simulink model "SHIP_DOWN_PT2000_matlab_2017"  (R2018b)
settings: Solver=ode8  StartTime=0.0  StopTime=2.5  RelTol=1e-3
undefined symbols (not defined in the file): Cout_c, Cout_r, Cvh_c, Cvh_r, dellay_f1, dellay_f2, dellay_f3, dellay_f4, dellay_f5, dellay_f6, DiscIntNeverNeededParam, f, L1_l, L1_r, Lvh_l, Lvh_r, R_out, Uout, Uvh
libraries: powerlib x92, simulink x18, simulink_extras x18, powerlib_meascontrol x13
(part 2 of 2)

== system SHIP_DOWN_PT2000_matlab_2017/Силовой блок 2/PWM4 ==
  Uz : Inport
  Data Type Conversion : DataTypeConversion  OutDataTypeStr=boolean
  Delay1 : Delay  DelayLength=dellay_f4  InitialCondition=0  UseCircularBuffer=on
  Logical Operator : Logic  Operator=NOT  AllPortsSameDT=off  OutDataTypeStr=boolean
  Relay1 : Relay  OnSwitchValue=0.01  OffSwitchValue=-0.01
  Repeating Sequence1 : simulink/Sources/Repeating Sequence  rep_seq_t="[0  (1/(2*f)) (1/f)]"  rep_seq_y=[0 1 0]
  S-R Flip-Flop : simulink_extras/Flip Flops/S-R Flip-Flop  initial_condition=0
  Sum : Sum  Inputs=+-
  Terminator : Terminator
  CH1 : Outport
  wires:
  S-R Flip-Flop/1 -> CH1/1
  Data Type Conversion/1 -> S-R Flip-Flop/1
  Logical Operator/1 -> S-R Flip-Flop/2
  Relay1/1 -> Logical Operator/1, Data Type Conversion/1
  Uz/1 -> Sum/1
  Sum/1 -> Relay1/1
  S-R Flip-Flop/2 -> Terminator/1
  Repeating Sequence1/1 -> Delay1/1
  Delay1/1 -> Sum/2

== system SHIP_DOWN_PT2000_matlab_2017/Силовой блок 2/PWM5 ==
  Uz : Inport
  Data Type Conversion : DataTypeConversion  OutDataTypeStr=boolean
  Delay1 : Delay  DelayLength=dellay_f5  InitialCondition=0  UseCircularBuffer=on
  Logical Operator : Logic  Operator=NOT  AllPortsSameDT=off  OutDataTypeStr=boolean
  Relay1 : Relay  OnSwitchValue=0.01  OffSwitchValue=-0.01
  Repeating Sequence1 : simulink/Sources/Repeating Sequence  rep_seq_t="[0  (1/(2*f)) (1/f)]"  rep_seq_y=[0 1 0]
  S-R Flip-Flop : simulink_extras/Flip Flops/S-R Flip-Flop  initial_condition=0
  Sum : Sum  Inputs=+-
  Terminator : Terminator
  CH1 : Outport
  wires:
  S-R Flip-Flop/1 -> CH1/1
  Data Type Conversion/1 -> S-R Flip-Flop/1
  Logical Operator/1 -> S-R Flip-Flop/2
  Relay1/1 -> Logical Operator/1, Data Type Conversion/1
  Uz/1 -> Sum/1
  Sum/1 -> Relay1/1
  S-R Flip-Flop/2 -> Terminator/1
  Repeating Sequence1/1 -> Delay1/1
  Delay1/1 -> Sum/2

== system SHIP_DOWN_PT2000_matlab_2017/Силовой блок 2/PWM6 ==
  Uz : Inport
  Data Type Conversion : DataTypeConversion  OutDataTypeStr=boolean
  Delay1 : Delay  DelayLength=dellay_f6  InitialCondition=0  UseCircularBuffer=on
  Logical Operator : Logic  Operator=NOT  AllPortsSameDT=off  OutDataTypeStr=boolean
  Relay1 : Relay  OnSwitchValue=0.01  OffSwitchValue=-0.01
  Repeating Sequence1 : simulink/Sources/Repeating Sequence  rep_seq_t="[0  (1/(2*f)) (1/f)]"  rep_seq_y=[0 1 0]
  S-R Flip-Flop : simulink_extras/Flip Flops/S-R Flip-Flop  initial_condition=0
  Sum : Sum  Inputs=+-
  Terminator : Terminator
  CH1 : Outport
  wires:
  S-R Flip-Flop/1 -> CH1/1
  Data Type Conversion/1 -> S-R Flip-Flop/1
  Logical Operator/1 -> S-R Flip-Flop/2
  Relay1/1 -> Logical Operator/1, Data Type Conversion/1
  Uz/1 -> Sum/1
  Sum/1 -> Relay1/1
  S-R Flip-Flop/2 -> Terminator/1
  Repeating Sequence1/1 -> Delay1/1
  Delay1/1 -> Sum/2

== system SHIP_DOWN_PT2000_matlab_2017/Силовой блок 3/PI I1 ==
  Zad : Inport
  OS : Inport  Port=2
  Discrete-Time Integrator2 : DiscreteIntegrator  SampleTime=-1  LimitOutput=on  UpperSaturationLimit=0.7  LowerSaturationLimit=0  ICPrevOutput=DiscIntNeverNeededParam  ICPrevScaledInput=DiscIntNeverNeededParam
  Proportional gain : Gain  Gain=0.01  SaturateOnIntegerOverflow=on  OutDataTypeStr=Inherit: Same as input  ParamDataTypeStr=Inherit: Same as input
  Proportional gain1 : Gain  Gain=0.2  SaturateOnIntegerOverflow=on  OutDataTypeStr=Inherit: Same as input  ParamDataTypeStr=Inherit: Same as input
  Saturation1 : Saturate  UpperLimit=0.7  LowerLimit=0
  Saturation2 : Saturate  UpperLimit=0.4  LowerLimit=0
  Scope1 : Scope  NumInputPorts=8
  Sum5 : Sum  Inputs=|+-  SaturateOnIntegerOverflow=on  InputSameDT=on  OutDataTypeStr=Inherit: Same as first input
  Sum6 : Sum  SaturateOnIntegerOverflow=on  InputSameDT=on  OutDataTypeStr=Inherit: Same as first input
  Out : Outport
  wires:
  Proportional gain/1 -> Saturation2/1
  Discrete-Time Integrator2/1 -> Sum6/2, Scope1/2  "Выход И РТ"
  OS/1 -> Scope1/5, Sum5/2  "Выходной ток"
  Zad/1 -> Scope1/6, Sum5/1  "Заданный ток"
  Sum5/1 -> Proportional gain1/1, Scope1/4, Proportional gain/1  "Рассогласование  РТ"
  Sum6/1 -> Saturation1/1
  Saturation1/1 -> Out/1, Scope1/1  "Выход РТ"
  Proportional gain1/1 -> Discrete-Time Integrator2/1
  Saturation2/1 -> Scope1/3, Sum6/1  "Выход РТ"

== system SHIP_DOWN_PT2000_matlab_2017/Силовой блок 3/PI I2 ==
  Zad : Inport
  OS : Inport  Port=2
  Discrete-Time Integrator2 : DiscreteIntegrator  SampleTime=-1  LimitOutput=on  UpperSaturationLimit=0.7  LowerSaturationLimit=0  ICPrevOutput=DiscIntNeverNeededParam  ICPrevScaledInput=DiscIntNeverNeededParam
  Proportional gain : Gain  Gain=0.01  SaturateOnIntegerOverflow=on  OutDataTypeStr=Inherit: Same as input  ParamDataTypeStr=Inherit: Same as input
  Proportional gain1 : Gain  Gain=0.2  SaturateOnIntegerOverflow=on  OutDataTypeStr=Inherit: Same as input  ParamDataTypeStr=Inherit: Same as input
  Saturation1 : Saturate  UpperLimit=0.7  LowerLimit=0
  Saturation2 : Saturate  UpperLimit=0.4  LowerLimit=0
  Scope1 : Scope  NumInputPorts=8
  Sum5 : Sum  Inputs=|+-  SaturateOnIntegerOverflow=on  InputSameDT=on  OutDataTypeStr=Inherit: Same as first input
  Sum6 : Sum  SaturateOnIntegerOverflow=on  InputSameDT=on  OutDataTypeStr=Inherit: Same as first input
  Out : Outport
  wires:
  Proportional gain/1 -> Saturation2/1
  Discrete-Time Integrator2/1 -> Sum6/2, Scope1/2  "Выход И РТ"
  OS/1 -> Scope1/5, Sum5/2  "Выходной ток"
  Zad/1 -> Scope1/6, Sum5/1  "Заданный ток"
  Sum5/1 -> Proportional gain1/1, Scope1/4, Proportional gain/1  "Рассогласование  РТ"
  Sum6/1 -> Saturation1/1
  Saturation1/1 -> Out/1, Scope1/1  "Выход РТ"
  Proportional gain1/1 -> Discrete-Time Integrator2/1
  Saturation2/1 -> Scope1/3, Sum6/1  "Выход РТ"

== system SHIP_DOWN_PT2000_matlab_2017/Силовой блок 3/PI I3 ==
  Zad : Inport
  OS : Inport  Port=2
  Discrete-Time Integrator2 : DiscreteIntegrator  SampleTime=-1  LimitOutput=on  UpperSaturationLimit=0.7  LowerSaturationLimit=0  ICPrevOutput=DiscIntNeverNeededParam  ICPrevScaledInput=DiscIntNeverNeededParam
  Proportional gain : Gain  Gain=0.01  SaturateOnIntegerOverflow=on  OutDataTypeStr=Inherit: Same as input  ParamDataTypeStr=Inherit: Same as input
  Proportional gain1 : Gain  Gain=0.2  SaturateOnIntegerOverflow=on  OutDataTypeStr=Inherit: Same as input  ParamDataTypeStr=Inherit: Same as input
  Saturation1 : Saturate  UpperLimit=0.7  LowerLimit=0
  Saturation2 : Saturate  UpperLimit=0.4  LowerLimit=0
  Scope1 : Scope  NumInputPorts=8
  Sum5 : Sum  Inputs=|+-  SaturateOnIntegerOverflow=on  InputSameDT=on  OutDataTypeStr=Inherit: Same as first input
  Sum6 : Sum  SaturateOnIntegerOverflow=on  InputSameDT=on  OutDataTypeStr=Inherit: Same as first input
  Out : Outport
  wires:
  Proportional gain/1 -> Saturation2/1
  Discrete-Time Integrator2/1 -> Sum6/2, Scope1/2  "Выход И РТ"
  OS/1 -> Scope1/5, Sum5/2  "Выходной ток"
  Zad/1 -> Scope1/6, Sum5/1  "Заданный ток"
  Sum5/1 -> Proportional gain1/1, Scope1/4, Proportional gain/1  "Рассогласование  РТ"
  Sum6/1 -> Saturation1/1
  Saturation1/1 -> Out/1, Scope1/1  "Выход РТ"
  Proportional gain1/1 -> Discrete-Time Integrator2/1
  Saturation2/1 -> Scope1/3, Sum6/1  "Выход РТ"

== system SHIP_DOWN_PT2000_matlab_2017/Силовой блок 3/PI I4 ==
  Zad : Inport
  OS : Inport  Port=2
  Discrete-Time Integrator2 : DiscreteIntegrator  SampleTime=-1  LimitOutput=on  UpperSaturationLimit=0.7  LowerSaturationLimit=0  ICPrevOutput=DiscIntNeverNeededParam  ICPrevScaledInput=DiscIntNeverNeededParam
  Proportional gain : Gain  Gain=0.01  SaturateOnIntegerOverflow=on  OutDataTypeStr=Inherit: Same as input  ParamDataTypeStr=Inherit: Same as input
  Proportional gain1 : Gain  Gain=0.2  SaturateOnIntegerOverflow=on  OutDataTypeStr=Inherit: Same as input  ParamDataTypeStr=Inherit: Same as input
  Saturation1 : Saturate  UpperLimit=0.7  LowerLimit=0
  Saturation2 : Saturate  UpperLimit=0.4  LowerLimit=0
  Scope1 : Scope  NumInputPorts=8
  Sum5 : Sum  Inputs=|+-  SaturateOnIntegerOverflow=on  InputSameDT=on  OutDataTypeStr=Inherit: Same as first input
  Sum6 : Sum  SaturateOnIntegerOverflow=on  InputSameDT=on  OutDataTypeStr=Inherit: Same as first input
  Out : Outport
  wires:
  Proportional gain/1 -> Saturation2/1
  Discrete-Time Integrator2/1 -> Sum6/2, Scope1/2  "Выход И РТ"
  OS/1 -> Scope1/5, Sum5/2  "Выходной ток"
  Zad/1 -> Scope1/6, Sum5/1  "Заданный ток"
  Sum5/1 -> Proportional gain1/1, Scope1/4, Proportional gain/1  "Рассогласование  РТ"
  Sum6/1 -> Saturation1/1
  Saturation1/1 -> Out/1, Scope1/1  "Выход РТ"
  Proportional gain1/1 -> Discrete-Time Integrator2/1
  Saturation2/1 -> Scope1/3, Sum6/1  "Выход РТ"

== system SHIP_DOWN_PT2000_matlab_2017/Силовой блок 3/PI I5 ==
  Zad : Inport
  OS : Inport  Port=2
  Discrete-Time Integrator2 : DiscreteIntegrator  SampleTime=-1  LimitOutput=on  UpperSaturationLimit=0.7  LowerSaturationLimit=0  ICPrevOutput=DiscIntNeverNeededParam  ICPrevScaledInput=DiscIntNeverNeededParam
  Proportional gain : Gain  Gain=0.01  SaturateOnIntegerOverflow=on  OutDataTypeStr=Inherit: Same as input  ParamDataTypeStr=Inherit: Same as input
  Proportional gain1 : Gain  Gain=0.2  SaturateOnIntegerOverflow=on  OutDataTypeStr=Inherit: Same as input  ParamDataTypeStr=Inherit: Same as input
  Saturation1 : Saturate  UpperLimit=0.7  LowerLimit=0
  Saturation2 : Saturate  UpperLimit=0.4  LowerLimit=0
  Scope1 : Scope  NumInputPorts=8
  Sum5 : Sum  Inputs=|+-  SaturateOnIntegerOverflow=on  InputSameDT=on  OutDataTypeStr=Inherit: Same as first input
  Sum6 : Sum  SaturateOnIntegerOverflow=on  InputSameDT=on  OutDataTypeStr=Inherit: Same as first input
  Out : Outport
  wires:
  Proportional gain/1 -> Saturation2/1
  Discrete-Time Integrator2/1 -> Sum6/2, Scope1/2  "Выход И РТ"
  OS/1 -> Scope1/5, Sum5/2  "Выходной ток"
  Zad/1 -> Scope1/6, Sum5/1  "Заданный ток"
  Sum5/1 -> Proportional gain1/1, Scope1/4, Proportional gain/1  "Рассогласование  РТ"
  Sum6/1 -> Saturation1/1
  Saturation1/1 -> Out/1, Scope1/1  "Выход РТ"
  Proportional gain1/1 -> Discrete-Time Integrator2/1
  Saturation2/1 -> Scope1/3, Sum6/1  "Выход РТ"

== system SHIP_DOWN_PT2000_matlab_2017/Силовой блок 3/PI I6 ==
  Zad : Inport
  OS : Inport  Port=2
  Discrete-Time Integrator2 : DiscreteIntegrator  SampleTime=-1  LimitOutput=on  UpperSaturationLimit=0.7  LowerSaturationLimit=0  ICPrevOutput=DiscIntNeverNeededParam  ICPrevScaledInput=DiscIntNeverNeededParam
  Proportional gain : Gain  Gain=0.01  SaturateOnIntegerOverflow=on  OutDataTypeStr=Inherit: Same as input  ParamDataTypeStr=Inherit: Same as input
  Proportional gain1 : Gain  Gain=0.2  SaturateOnIntegerOverflow=on  OutDataTypeStr=Inherit: Same as input  ParamDataTypeStr=Inherit: Same as input
  Saturation1 : Saturate  UpperLimit=0.7  LowerLimit=0
  Saturation2 : Saturate  UpperLimit=0.4  LowerLimit=0
  Scope1 : Scope  NumInputPorts=8
  Sum5 : Sum  Inputs=|+-  SaturateOnIntegerOverflow=on  InputSameDT=on  OutDataTypeStr=Inherit: Same as first input
  Sum6 : Sum  SaturateOnIntegerOverflow=on  InputSameDT=on  OutDataTypeStr=Inherit: Same as first input
  Out : Outport
  wires:
  Proportional gain/1 -> Saturation2/1
  Discrete-Time Integrator2/1 -> Sum6/2, Scope1/2  "Выход И РТ"
  OS/1 -> Scope1/5, Sum5/2  "Выходной ток"
  Zad/1 -> Scope1/6, Sum5/1  "Заданный ток"
  Sum5/1 -> Proportional gain1/1, Scope1/4, Proportional gain/1  "Рассогласование  РТ"
  Sum6/1 -> Saturation1/1
  Saturation1/1 -> Out/1, Scope1/1  "Выход РТ"
  Proportional gain1/1 -> Discrete-Time Integrator2/1
  Saturation2/1 -> Scope1/3, Sum6/1  "Выход РТ"

== system SHIP_DOWN_PT2000_matlab_2017/Силовой блок 3/PWM1 ==
  Uz : Inport
  Data Type Conversion : DataTypeConversion  OutDataTypeStr=boolean
  Delay1 : Delay  DelayLength=dellay_f1  InitialCondition=0  UseCircularBuffer=on
  Logical Operator : Logic  Operator=NOT  AllPortsSameDT=off  OutDataTypeStr=boolean
  Relay1 : Relay  OnSwitchValue=0.01  OffSwitchValue=-0.01
  Repeating Sequence1 : simulink/Sources/Repeating Sequence  rep_seq_t="[0  (1/(2*f)) (1/f)]"  rep_seq_y=[0 1 0]
  S-R Flip-Flop : simulink_extras/Flip Flops/S-R Flip-Flop  initial_condition=0
  Sum : Sum  Inputs=+-
  Terminator : Terminator
  CH1 : Outport
  wires:
  S-R Flip-Flop/1 -> CH1/1
  Data Type Conversion/1 -> S-R Flip-Flop/1
  Logical Operator/1 -> S-R Flip-Flop/2
  Relay1/1 -> Logical Operator/1, Data Type Conversion/1
  Uz/1 -> Sum/1
  Sum/1 -> Relay1/1
  S-R Flip-Flop/2 -> Terminator/1
  Repeating Sequence1/1 -> Delay1/1
  Delay1/1 -> Sum/2

== system SHIP_DOWN_PT2000_matlab_2017/Силовой блок 3/PWM2 ==
  Uz : Inport
  Data Type Conversion : DataTypeConversion  OutDataTypeStr=boolean
  Delay1 : Delay  DelayLength=dellay_f2  InitialCondition=0  UseCircularBuffer=on
  Logical Operator : Logic  Operator=NOT  AllPortsSameDT=off  OutDataTypeStr=boolean
  Relay1 : Relay  OnSwitchValue=0.01  OffSwitchValue=-0.01
  Repeating Sequence1 : simulink/Sources/Repeating Sequence  rep_seq_t="[0  (1/(2*f)) (1/f)]"  rep_seq_y=[0 1 0]
  S-R Flip-Flop : simulink_extras/Flip Flops/S-R Flip-Flop  initial_condition=0
  Sum : Sum  Inputs=+-
  Terminator : Terminator
  CH1 : Outport
  wires:
  S-R Flip-Flop/1 -> CH1/1
  Data Type Conversion/1 -> S-R Flip-Flop/1
  Logical Operator/1 -> S-R Flip-Flop/2
  Relay1/1 -> Logical Operator/1, Data Type Conversion/1
  Uz/1 -> Sum/1
  Sum/1 -> Relay1/1
  S-R Flip-Flop/2 -> Terminator/1
  Repeating Sequence1/1 -> Delay1/1
  Delay1/1 -> Sum/2

== system SHIP_DOWN_PT2000_matlab_2017/Силовой блок 3/PWM3 ==
  Uz : Inport
  Data Type Conversion : DataTypeConversion  OutDataTypeStr=boolean
  Delay1 : Delay  DelayLength=dellay_f3  InitialCondition=0  UseCircularBuffer=on
  Logical Operator : Logic  Operator=NOT  AllPortsSameDT=off  OutDataTypeStr=boolean
  Relay1 : Relay  OnSwitchValue=0.01  OffSwitchValue=-0.01
  Repeating Sequence1 : simulink/Sources/Repeating Sequence  rep_seq_t="[0  (1/(2*f)) (1/f)]"  rep_seq_y=[0 1 0]
  S-R Flip-Flop : simulink_extras/Flip Flops/S-R Flip-Flop  initial_condition=0
  Sum : Sum  Inputs=+-
  Terminator : Terminator
  CH1 : Outport
  wires:
  S-R Flip-Flop/1 -> CH1/1
  Data Type Conversion/1 -> S-R Flip-Flop/1
  Logical Operator/1 -> S-R Flip-Flop/2
  Relay1/1 -> Logical Operator/1, Data Type Conversion/1
  Uz/1 -> Sum/1
  Sum/1 -> Relay1/1
  S-R Flip-Flop/2 -> Terminator/1
  Repeating Sequence1/1 -> Delay1/1
  Delay1/1 -> Sum/2

== system SHIP_DOWN_PT2000_matlab_2017/Силовой блок 3/PWM4 ==
  Uz : Inport
  Data Type Conversion : DataTypeConversion  OutDataTypeStr=boolean
  Delay1 : Delay  DelayLength=dellay_f4  InitialCondition=0  UseCircularBuffer=on
  Logical Operator : Logic  Operator=NOT  AllPortsSameDT=off  OutDataTypeStr=boolean
  Relay1 : Relay  OnSwitchValue=0.01  OffSwitchValue=-0.01
  Repeating Sequence1 : simulink/Sources/Repeating Sequence  rep_seq_t="[0  (1/(2*f)) (1/f)]"  rep_seq_y=[0 1 0]
  S-R Flip-Flop : simulink_extras/Flip Flops/S-R Flip-Flop  initial_condition=0
  Sum : Sum  Inputs=+-
  Terminator : Terminator
  CH1 : Outport
  wires:
  S-R Flip-Flop/1 -> CH1/1
  Data Type Conversion/1 -> S-R Flip-Flop/1
  Logical Operator/1 -> S-R Flip-Flop/2
  Relay1/1 -> Logical Operator/1, Data Type Conversion/1
  Uz/1 -> Sum/1
  Sum/1 -> Relay1/1
  S-R Flip-Flop/2 -> Terminator/1
  Repeating Sequence1/1 -> Delay1/1
  Delay1/1 -> Sum/2

== system SHIP_DOWN_PT2000_matlab_2017/Силовой блок 3/PWM5 ==
  Uz : Inport
  Data Type Conversion : DataTypeConversion  OutDataTypeStr=boolean
  Delay1 : Delay  DelayLength=dellay_f5  InitialCondition=0  UseCircularBuffer=on
  Logical Operator : Logic  Operator=NOT  AllPortsSameDT=off  OutDataTypeStr=boolean
  Relay1 : Relay  OnSwitchValue=0.01  OffSwitchValue=-0.01
  Repeating Sequence1 : simulink/Sources/Repeating Sequence  rep_seq_t="[0  (1/(2*f)) (1/f)]"  rep_seq_y=[0 1 0]
  S-R Flip-Flop : simulink_extras/Flip Flops/S-R Flip-Flop  initial_condition=0
  Sum : Sum  Inputs=+-
  Terminator : Terminator
  CH1 : Outport
  wires:
  S-R Flip-Flop/1 -> CH1/1
  Data Type Conversion/1 -> S-R Flip-Flop/1
  Logical Operator/1 -> S-R Flip-Flop/2
  Relay1/1 -> Logical Operator/1, Data Type Conversion/1
  Uz/1 -> Sum/1
  Sum/1 -> Relay1/1
  S-R Flip-Flop/2 -> Terminator/1
  Repeating Sequence1/1 -> Delay1/1
  Delay1/1 -> Sum/2

== system SHIP_DOWN_PT2000_matlab_2017/Силовой блок 3/PWM6 ==
  Uz : Inport
  Data Type Conversion : DataTypeConversion  OutDataTypeStr=boolean
  Delay1 : Delay  DelayLength=dellay_f6  InitialCondition=0  UseCircularBuffer=on
  Logical Operator : Logic  Operator=NOT  AllPortsSameDT=off  OutDataTypeStr=boolean
  Relay1 : Relay  OnSwitchValue=0.01  OffSwitchValue=-0.01
  Repeating Sequence1 : simulink/Sources/Repeating Sequence  rep_seq_t="[0  (1/(2*f)) (1/f)]"  rep_seq_y=[0 1 0]
  S-R Flip-Flop : simulink_extras/Flip Flops/S-R Flip-Flop  initial_condition=0
  Sum : Sum  Inputs=+-
  Terminator : Terminator
  CH1 : Outport
  wires:
  S-R Flip-Flop/1 -> CH1/1
  Data Type Conversion/1 -> S-R Flip-Flop/1
  Logical Operator/1 -> S-R Flip-Flop/2
  Relay1/1 -> Logical Operator/1, Data Type Conversion/1
  Uz/1 -> Sum/1
  Sum/1 -> Relay1/1
  S-R Flip-Flop/2 -> Terminator/1
  Repeating Sequence1/1 -> Delay1/1
  Delay1/1 -> Sum/2
